simulink model "mm10s2"  (Simulink 8.1)
settings: Solver=ode45  StartTime=0.0  StopTime=10  FixedStep=T  RelTol=1e-3
values from neighbouring files (symbols this model uses):
  Alpha = fliplr(transpose(AlphaBeta(1:2)))    [mm10s2_init.m]    (also in mm3679_init.m = fliplr(transpose(M(1:2))))
  Beta = fliplr(transpose(AlphaBeta(3:4)))    [mm10s2_init.m]    (also in mm3679_init.m = fliplr(transpose(M(3:4))))
  QAz = conv(Alpha, Am)    [mm10s2_init.m]
  QBz = conv(H1, conv(F, Bm))    [mm10s2_init.m]
  T = 0.5    [mm10s2_init.m]    (also in mm3679_init.m = 1)
libraries: simulink x1
settings Model: Creator=jmahler  LastModifiedBy=jmahler
settings DataIOCC: SignalLoggingSaveFormat=Dataset
settings OptimizationCC: ExpressionDepthLimit=128
settings DebuggingCC: SolverPrmCheckMsg=none  FcnCallInpInsideContextMsg=EnableAllAsError
settings GRTTargetCC: CombineOutputUpdateFcns=on  GRTInterface=off

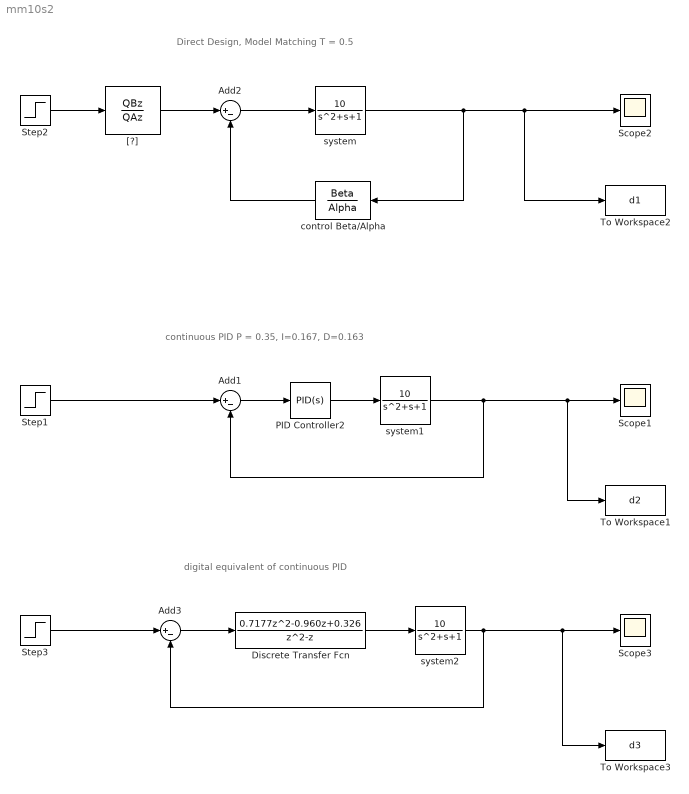
== system mm10s2 ==
  note: Direct Design, Model Matching
      | T = 0.5
  note: continuous PID
      | P = 0.35, I=0.167, D=0.163
  note: digital equivalent of continuous PID
  Add1 : Sum  Inputs=|+-
  Add2 : Sum  Inputs=|+-
  Add3 : Sum  Inputs=|+-
  Discrete Transfer Fcn : DiscreteTransferFcn  Numerator=[0.7177 -0.960 0.326]  Denominator=[1 -1 0]  SampleTime=T
  PID Controller2 : simulink/Continuous/PID Controller  Controller=PID  TimeDomain=Continuous-time  SampleTime=1  IntegratorMethod=Forward Euler  FilterMethod=Forward Euler  Form=Parallel  P=0.35  I=0.167  D=0.163  N=100  InitialConditionSource=internal  InitialConditionForIntegrator=0  InitialConditionForFilter=0  ExternalReset=none  LimitOutput=off  UpperSaturationLimit=inf  LowerSaturationLimit=-inf  LinearizeAsGain=on  AntiWindupMode=none  Kb=1  TrackingMode=off  Kt=1  PParamMin=[]  PParamMax=[]  IParamMin=[]  IParamMax=[]  DParamMin=[]  DParamMax=[]  NParamMin=[]  NParamMax=[]  KbParamMin=[]  KbParamMax=[]  KtParamMin=[]  KtParamMax=[]  POutMin=[]  POutMax=[]  IOutMin=[]  IOutMax=[]  DOutMin=[]  DOutMax=[]  NOutMin=[]  NOutMax=[]  KbOutMin=[]  KbOutMax=[]  KtOutMin=[]  KtOutMax=[]  IntegratorOutMin=[]  IntegratorOutMax=[]  FilterOutMin=[]  FilterOutMax=[]  SumOutMin=[]  SumOutMax=[]  SumI1OutMin=[]  SumI1OutMax=[]  SumI2OutMin=[]  SumI2OutMax=[]  SumI3OutMin=[]  SumI3OutMax=[]  SumDOutMin=[]  SumDOutMax=[]  SaturationOutMin=[]  SaturationOutMax=[]  IntegratorContinuousStateAttributes=''  IntegratorStateMustResolveToSignalObject=off  IntegratorRTWStateStorageClass=Auto  FilterContinuousStateAttributes=''  FilterStateMustResolveToSignalObject=off  FilterRTWStateStorageClass=Auto
  Scope1 : Scope
  Scope2 : Scope
  Scope3 : Scope
      settings: SaveName=ScopeData2
  Step1 : Step  Time=0  SampleTime=0
  Step2 : Step  Time=0  SampleTime=0
  Step3 : Step  Time=0  SampleTime=0
  To Workspace1 : ToWorkspace  VariableName=d2  SampleTime=-1  SaveFormat=Timeseries
  To Workspace2 : ToWorkspace  VariableName=d1  SampleTime=-1  SaveFormat=Timeseries
  To Workspace3 : ToWorkspace  VariableName=d3  SampleTime=-1  SaveFormat=Timeseries
  "[?]" : DiscreteTransferFcn  Numerator=QBz  Denominator=QAz  SampleTime=T
  control Beta/Alpha : DiscreteTransferFcn  Numerator=Beta  Denominator=Alpha  SampleTime=T
  system : TransferFcn  Numerator=[10]  Denominator=[1 1 1]
  system1 : TransferFcn  Numerator=[10]  Denominator=[1 1 1]
  system2 : TransferFcn  Numerator=[10]  Denominator=[1 1 1]
  wires:
  control Beta/Alpha/1 -> Add2/2
  Add2/1 -> system/1
  system/1 -> control Beta/Alpha/1, Scope2/1, To Workspace2/1
  Step2/1 -> "[?]"/1
  "[?]"/1 -> Add2/1
  system1/1 -> To Workspace1/1, Scope1/1, Add1/2
  Step1/1 -> Add1/1
  PID Controller2/1 -> system1/1
  Add1/1 -> PID Controller2/1
  system2/1 -> To Workspace3/1, Scope3/1, Add3/2
  Step3/1 -> Add3/1
  Discrete Transfer Fcn/1 -> system2/1
  Add3/1 -> Discrete Transfer Fcn/1
